simulink model "EcoSIM3_P2_C2_WIP"  (R2014b)
settings: Solver=ode1  SolverMode=SingleTasking  StartTime=0.0  StopTime=4  FixedStep=0.01  RelTol=1e-3
PostLoadFcn:
  | %, if any(exist('dsrtsu_mdlpostloadfcn', 'file') == [2, 3, 6]), try dsrtsu_mdlpostloadfcn('Execute', bdroot); catch fprintf('Error in PostLoadFcn (dsrtsu_mdlpostloadfcn) for model "%s":\n %s\n', bdroot, lasterr); end, end,
InitFcn:
  | tic
  | %Startup_EcoSIM
undefined symbols (not defined in the file or in its folder): canChannel, Controls, DriveCycles, Driver, EM_EFF_MAP, EM_PwrLoss_MAP, EngPwr, EngSpd, EngTrq, Glbl, Overwritten_Mode, Plants, Power, sigbuilder_block, Torque, Trialmap, Veh_Dynamics
libraries: simulink x135, canmsglib x113, fl_lib x104, canlib x89, nesl_utility x56, sdl_lib x29, dspsigops x6, dspswit3 x5, dspstat3 x2, commnoisgen2 x1, dspfdesign x1
(part 15 of 21)

== system EcoSIM3_P2_C2_WIP/Supervisory Controller/Supervisory_IO/VNT Vector/CAN Rx/GCM ==
  Bus Creator7 : BusCreator  Inputs=3
  CAN Receive9 : canlib/CAN Receive  BlockHandle=18097.0002  DeviceMenu=Vector Virtual 1 (Channel 1)  Device=Vector Virtual 1 (Channel 1)  ObjConstructor=canChannel('Vector', 'Virtual 1', 1)  EnableStandardIDsFilter=off  StandardIDs=52  EnableExtendedIDsFilter=off  ExtendedIDs=0  SampleTime=0.01  MsgsPerTimestep=1  StdIDsCombo=Allow only  ExtIDsCombo=Block all  InternalFilterUpdateStatus=on
  CAN Unpack9 : canmsglib/CAN Unpack  CANdbFile=C:\Box Sync\EcoCAR 3\SMS\EcoSIM3_P2_C2\MIL\Final_DBC\EcoCAR3_Controls_Development.dbc  MsgList=GCM_Transmit_MSG052  MsgName=GCM_Transmit_MSG052  MsgIDType=Standard (11-bit identifier)  MsgIdentifier=52  MsgLength=2  SignalInfo=GCM_Heartbeat$2$5$2$2$1$0$1$0$0$31$#GCM_Reported_Gear$13$3$2$1$1$0$1$3$-1$6$#Shift_Complete$1$1$2$2$1$0$1$0$0$1$#charge_mode_request$7$1$2$2$1$0$1$0$0$1$#  NSignals=4  IDPort=off  TimestampPort=off  ErrorPort=off  RemotePort=off  LengthPort=off  StatusPort=off  StartBits=str2num('[int32(2);int32(13);int32(1);int32(7)]')  SignalSizes=str2num('[int32(5);int32(3);int32(1);int32(1)]')  ByteOrders=str2num('[int32(2);int32(2);int32(2);int32(2)]')  DataTypes=str2num('[int32(2);int32(1);int32(2);int32(2)]')  MultiplexTypes=str2num('[int32(1);int32(1);int32(1);int32(1)]')  MultiplexValues=str2num('[double(0);double(0);double(0);double(0)]')  Factors=str2num('[double(1);double(1);double(1);double(1)]')  Offsets=str2num('[double(0);double(3);double(0);double(0)]')  Minimums=str2num('[double(0);double(-1);double(0);double(0)]')  Maximums=str2num('[double(31);double(6);double(1);double(1)]')
      settings: DataFormat=CANdb specified signals
  Terminator10 : Terminator
  FromGCM : Outport
  wires:
  CAN Receive9/2 -> CAN Unpack9/1
  CAN Receive9/1 -> Terminator10/1
  CAN Unpack9/4 -> Bus Creator7/3  "charge_mode_request"
  Bus Creator7/1 -> FromGCM/1  "GCM_CAN_Out"
  CAN Unpack9/3 -> Bus Creator7/2  "Shift_Complete"
  CAN Unpack9/2 -> Bus Creator7/1  "GCM_Reported_Gear"

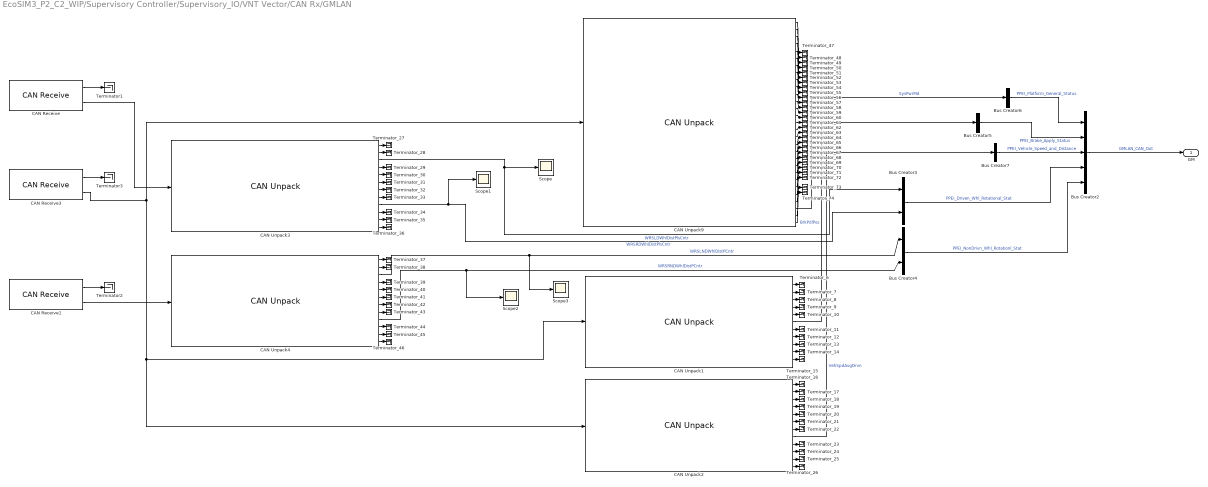
== system EcoSIM3_P2_C2_WIP/Supervisory Controller/Supervisory_IO/VNT Vector/CAN Rx/GMLAN ==
  Bus Creator2 : BusCreator  Inputs=5
  Bus Creator3 : BusCreator  Inputs=2
  Bus Creator4 : BusCreator  Inputs=2
  Bus Creator5 : BusCreator  Inputs=1
  Bus Creator6 : BusCreator  Inputs=1
  Bus Creator7 : BusCreator  Inputs=1
  CAN Receive : canlib/CAN Receive  BlockHandle=18114.0005  DeviceMenu=Kvaser Virtual 1 (Channel 1)  Device=Vector Virtual 1 (Channel 1)  ObjConstructor=canChannel('Vector', 'Virtual 1', 1)  EnableStandardIDsFilter=off  StandardIDs=193  EnableExtendedIDsFilter=off  ExtendedIDs=0  SampleTime=0.01  MsgsPerTimestep=all  StdIDsCombo=Allow only  ExtIDsCombo=Allow all  InternalFilterUpdateStatus=on
  CAN Receive1 : canlib/CAN Receive  BlockHandle=18115.0001  DeviceMenu=Kvaser Virtual 1 (Channel 1)  Device=Vector Virtual 1 (Channel 1)  ObjConstructor=canChannel('Vector', 'Virtual 1', 1)  EnableStandardIDsFilter=off  StandardIDs=197  EnableExtendedIDsFilter=off  ExtendedIDs=0  SampleTime=0.01  MsgsPerTimestep=all  StdIDsCombo=Allow only  ExtIDsCombo=Allow all  InternalFilterUpdateStatus=on
  CAN Receive3 : canlib/CAN Receive  BlockHandle=18116.0001  DeviceMenu=Kvaser Virtual 1 (Channel 1)  Device=Vector Virtual 1 (Channel 1)  ObjConstructor=canChannel('Vector', 'Virtual 1', 1)  EnableStandardIDsFilter=off  StandardIDs=[193 197 241 497 1001]  EnableExtendedIDsFilter=off  ExtendedIDs=0  SampleTime=0.01  MsgsPerTimestep=1  StdIDsCombo=Allow only  ExtIDsCombo=Block all  InternalFilterUpdateStatus=on
  CAN Unpack1 : canmsglib/CAN Unpack  CANdbFile=C:\Users\EcoCAR_HIL\Documents\Khanna\EcoSIM3_P1_0_PHEV_TCU\Final_DBC\GlobalAHS_anon GM CONFIDENTIAL.dbc  MsgList=PPEI_Brake_Apply_Status  MsgName=PPEI_Brake_Apply_Status  MsgIDType=Standard (11-bit identifier)  MsgIdentifier=241  MsgLength=6  SignalInfo=BrkAppSnsrHmPosLrnd$30$1$2$2$1$0$1$0$0$1$#BrkPdlChkData$40$17$2$2$1$0$1$0$0$131071$#BrkPdlInTrvPrt$2$2$2$2$1$0$1$0$0$3$#BrkPdlModTrvl$6$1$2$2$1$0$1$0$0$1$#BrkPdlModTrvlV$7$1$2$2$1$0$1$0$0$1$#BrkPdlPos$8$8$2$2$1$0$3.921570e-01$0$0$1.000000e+02$#BrkPdlPosGrad$16$8$2$1$1$0$40$0$-5120$5080$#BrkPedPosAlvRolngCnt$4$2$2$2$1$0$1$0$0$3$#BrkPedTrvlAchvd$1$1$2$2$1$0$1$0$0$1$#BrkPedTrvlAchvdV$0$1$2$2$1$0$1$0$0$1$#NotEventStat$28$2$2$2$1$0$1$0$0$3$#  NSignals=11  IDPort=off  TimestampPort=off  ErrorPort=off  RemotePort=off  LengthPort=off  StatusPort=off  StartBits=str2num('[int32(30);int32(40);int32(2);int32(6);int32(7);int32(8);int32(16);int32(4);int32(1);int32(0);int32(28)]')  SignalSizes=str2num('[int32(1);int32(17);int32(2);int32(1);int32(1);int32(8);int32(8);int32(2);int32(1);int32(1);int32(2)]')  ByteOrders=str2num('[int32(2);int32(2);int32(2);int32(2);int32(2);int32(2);int32(2);int32(2);int32(2);int32(2);int32(2)]')  DataTypes=str2num('[int32(2);int32(2);int32(2);int32(2);int32(2);int32(2);int32(1);int32(2);int32(2);int32(2);int32(2)]')  MultiplexTypes=str2num('[int32(1);int32(1);int32(1);int32(1);int32(1);int32(1);int32(1);int32(1);int32(1);int32(1);int32(1)]')  MultiplexValues=str2num('[double(0);double(0);double(0);double(0);double(0);double(0);double(0);double(0);double(0);double(0);double(0)]')  Factors=str2num('[double(1);double(1);double(1);double(1);double(1);double(3.921570e-01);double(40);double(1);double(1);double(1);double(1)]')  Offsets=str2num('[double(0);double(0);double(0);double(0);double(0);double(0);double(0);double(0);double(0);double(0);double(0)]')  Minimums=str2num('[double(0);double(0);double(0);double(0);double(0);double(0);double(-5120);double(0);double(0);double(0);double(0)]')  Maximums=str2num('[double(1);double(131071);double(3);double(1);double(1);double(1.000000e+02);double(5080);double(3);double(1);double(1);double(3)]')
      settings: DataFormat=CANdb specified signals
  CAN Unpack2 : canmsglib/CAN Unpack  CANdbFile=C:\Users\EcoCAR_HIL\Documents\Khanna\EcoSIM3_P1_0_PHEV_TCU\Final_DBC\GlobalAHS_anon GM CONFIDENTIAL.dbc  MsgList=PPEI_Vehicle_Speed_and_Distance  MsgName=PPEI_Vehicle_Speed_and_Distance  MsgIDType=Standard (11-bit identifier)  MsgIdentifier=1001  MsgLength=8  SignalInfo=DistRollCntAvgDrvn$24$13$2$2$1$0$1.250000e-01$0$0$1.023875e+03$#DistRollCntAvgDrvnSrc$55$1$2$2$1$0$1$0$0$1$#DistRollCntAvgDrvnV$22$1$2$2$1$0$1$0$0$1$#DstRolCntAvNDrRstOc$53$1$2$2$1$0$1$0$0$1$#DstRolCntAvgDrnRstOc$21$1$2$2$1$0$1$0$0$1$#DstRolCntAvgNonDrvn$56$13$2$2$1$0$1.250000e-01$0$0$1.023875e+03$#DstRolCntAvgNonDrvnV$54$1$2$2$1$0$1$0$0$1$#VehSpdAvgDrvn$8$15$2$2$1$0$1.562500e-02$0$0$5.119844e+02$#VehSpdAvgDrvnSrc$23$1$2$2$1$0$1$0$0$1$#VehSpdAvgDrvnV$7$1$2$2$1$0$1$0$0$1$#VehSpdAvgNDrvn$40$15$2$2$1$0$1.562500e-02$0$0$5.119844e+02$#VehSpdAvgNDrvnV$39$1$2$2$1$0$1$0$0$1$#  NSignals=12  IDPort=off  TimestampPort=off  ErrorPort=off  RemotePort=off  LengthPort=off  StatusPort=off  StartBits=str2num('[int32(24);int32(55);int32(22);int32(53);int32(21);int32(56);int32(54);int32(8);int32(23);int32(7);int32(40);int32(39)]')  SignalSizes=str2num('[int32(13);int32(1);int32(1);int32(1);int32(1);int32(13);int32(1);int32(15);int32(1);int32(1);int32(15);int32(1)]')  ByteOrders=str2num('[int32(2);int32(2);int32(2);int32(2);int32(2);int32(2);int32(2);int32(2);int32(2);int32(2);int32(2);int32(2)]')  DataTypes=str2num('[int32(2);int32(2);int32(2);int32(2);int32(2);int32(2);int32(2);int32(2);int32(2);int32(2);int32(2);int32(2)]')  MultiplexTypes=str2num('[int32(1);int32(1);int32(1);int32(1);int32(1);int32(1);int32(1);int32(1);int32(1);int32(1);int32(1);int32(1)]')  MultiplexValues=str2num('[double(0);double(0);double(0);double(0);double(0);double(0);double(0);double(0);double(0);double(0);double(0);double(0)]')  Factors=str2num('[double(1.250000e-01);double(1);double(1);double(1);double(1);double(1.250000e-01);double(1);double(1.562500e-02);double(1);double(1);double(1.562500e-02);double(1)]')  Offsets=str2num('[double(0);double(0);double(0);double(0);double(0);double(0);double(0);double(0);double(0);double(0);double(0);double(0)]')  Minimums=str2num('[double(0);double(0);double(0);double(0);double(0);double(0);double(0);double(0);double(0);double(0);double(0);double(0)]')  Maximums=str2num('[double(1.023875e+03);double(1);double(1);double(1);double(1);double(1.023875e+03);double(1);double(5.119844e+02);double(1);double(1);double(5.119844e+02);double(1)]')
      settings: DataFormat=CANdb specified signals
  CAN Unpack3 : canmsglib/CAN Unpack  CANdbFile=C:\Users\EcoCAR_HIL\Documents\Khanna\EcoSIM3_P1_0_PHEV_TCU\Final_DBC\GlobalAHS_anon GM CONFIDENTIAL.dbc  MsgList=PPEI_Driven_Whl_Rotational_Stat  MsgName=PPEI_Driven_Whl_Rotational_Stat  MsgIDType=Standard (11-bit identifier)  MsgIdentifier=193  MsgLength=8  SignalInfo=WRSLDSeqNum$4$2$2$2$1$0$1$0$0$3$#WRSLDWhlDisTpRC$6$2$2$2$1$0$1$0$0$3$#WRSLDWhlDistPlsCntr$8$10$2$2$1$0$1$0$0$1023$#WRSLDWhlDistTmstm$24$16$2$2$1$0$1$0$0$65535$#WRSLDWhlDistVal$2$1$2$2$1$0$1$0$0$1$#WRSLDWhlRotStatRst$3$1$2$2$1$0$1$0$0$1$#WRSRDSeqNum$36$2$2$2$1$0$1$0$0$3$#WRSRDWhlDisTpRC$38$2$2$2$1$0$1$0$0$3$#WRSRDWhlDistPlsCntr$40$10$2$2$1$0$1$0$0$1023$#WRSRDWhlDistTmstm$56$16$2$2$1$0$1$0$0$65535$#WRSRDWhlDistVal$34$1$2$2$1$0$1$0$0$1$#WRSRDWhlRotStatRst$35$1$2$2$1$0$1$0$0$1$#  NSignals=12  IDPort=off  TimestampPort=off  ErrorPort=off  RemotePort=off  LengthPort=off  StatusPort=off  StartBits=str2num('[int32(4);int32(6);int32(8);int32(24);int32(2);int32(3);int32(36);int32(38);int32(40);int32(56);int32(34);int32(35)]')  SignalSizes=str2num('[int32(2);int32(2);int32(10);int32(16);int32(1);int32(1);int32(2);int32(2);int32(10);int32(16);int32(1);int32(1)]')  ByteOrders=str2num('[int32(2);int32(2);int32(2);int32(2);int32(2);int32(2);int32(2);int32(2);int32(2);int32(2);int32(2);int32(2)]')  DataTypes=str2num('[int32(2);int32(2);int32(2);int32(2);int32(2);int32(2);int32(2);int32(2);int32(2);int32(2);int32(2);int32(2)]')  MultiplexTypes=str2num('[int32(1);int32(1);int32(1);int32(1);int32(1);int32(1);int32(1);int32(1);int32(1);int32(1);int32(1);int32(1)]')  MultiplexValues=str2num('[double(0);double(0);double(0);double(0);double(0);double(0);double(0);double(0);double(0);double(0);double(0);double(0)]')  Factors=str2num('[double(1);double(1);double(1);double(1);double(1);double(1);double(1);double(1);double(1);double(1);double(1);double(1)]')  Offsets=str2num('[double(0);double(0);double(0);double(0);double(0);double(0);double(0);double(0);double(0);double(0);double(0);double(0)]')  Minimums=str2num('[double(0);double(0);double(0);double(0);double(0);double(0);double(0);double(0);double(0);double(0);double(0);double(0)]')  Maximums=str2num('[double(3);double(3);double(1023);double(65535);double(1);double(1);double(3);double(3);double(1023);double(65535);double(1);double(1)]')
      settings: DataFormat=CANdb specified signals
  CAN Unpack4 : canmsglib/CAN Unpack  CANdbFile=C:\Users\EcoCAR_HIL\Documents\Khanna\EcoSIM3_P1_0_PHEV_TCU\Final_DBC\GlobalAHS_anon GM CONFIDENTIAL.dbc  MsgList=PPEI_NonDrivn_Whl_Rotationl_Stat  MsgName=PPEI_NonDrivn_Whl_Rotationl_Stat  MsgIDType=Standard (11-bit identifier)  MsgIdentifier=197  MsgLength=8  SignalInfo=WRSLNDSeqNum$4$2$2$2$1$0$1$0$0$3$#WRSLNDWhlDisTpRC$6$2$2$2$1$0$1$0$0$3$#WRSLNDWhlDistPCntr$8$10$2$2$1$0$1$0$0$1023$#WRSLNDWhlDistTstm$24$16$2$2$1$0$1$0$0$65535$#WRSLNDWhlDistVal$2$1$2$2$1$0$1$0$0$1$#WRSLNDWhlRotStRst$3$1$2$2$1$0$1$0$0$1$#WRSRNDSeqNum$36$2$2$2$1$0$1$0$0$3$#WRSRNDWhlDisTpRC$38$2$2$2$1$0$1$0$0$3$#WRSRNDWhlDistPCntr$40$10$2$2$1$0$1$0$0$1023$#WRSRNDWhlDistTstm$56$16$2$2$1$0$1$0$0$65535$#WRSRNDWhlDistVal$34$1$2$2$1$0$1$0$0$1$#WRSRNDWhlRotStRst$35$1$2$2$1$0$1$0$0$1$#  NSignals=12  IDPort=off  TimestampPort=off  ErrorPort=off  RemotePort=off  LengthPort=off  StatusPort=off  StartBits=str2num('[int32(4);int32(6);int32(8);int32(24);int32(2);int32(3);int32(36);int32(38);int32(40);int32(56);int32(34);int32(35)]')  SignalSizes=str2num('[int32(2);int32(2);int32(10);int32(16);int32(1);int32(1);int32(2);int32(2);int32(10);int32(16);int32(1);int32(1)]')  ByteOrders=str2num('[int32(2);int32(2);int32(2);int32(2);int32(2);int32(2);int32(2);int32(2);int32(2);int32(2);int32(2);int32(2)]')  DataTypes=str2num('[int32(2);int32(2);int32(2);int32(2);int32(2);int32(2);int32(2);int32(2);int32(2);int32(2);int32(2);int32(2)]')  MultiplexTypes=str2num('[int32(1);int32(1);int32(1);int32(1);int32(1);int32(1);int32(1);int32(1);int32(1);int32(1);int32(1);int32(1)]')  MultiplexValues=str2num('[double(0);double(0);double(0);double(0);double(0);double(0);double(0);double(0);double(0);double(0);double(0);double(0)]')  Factors=str2num('[double(1);double(1);double(1);double(1);double(1);double(1);double(1);double(1);double(1);double(1);double(1);double(1)]')  Offsets=str2num('[double(0);double(0);double(0);double(0);double(0);double(0);double(0);double(0);double(0);double(0);double(0);double(0)]')  Minimums=str2num('[double(0);double(0);double(0);double(0);double(0);double(0);double(0);double(0);double(0);double(0);double(0);double(0)]')  Maximums=str2num('[double(3);double(3);double(1023);double(65535);double(1);double(1);double(3);double(3);double(1023);double(65535);double(1);double(1)]')
      settings: DataFormat=CANdb specified signals
  CAN Unpack9 : canmsglib/CAN Unpack  CANdbFile=C:\Users\EcoCAR_HIL\Documents\Khanna\EcoSIM3_P1_0_PHEV_TCU\Final_DBC\GlobalAHS_anon GM CONFIDENTIAL.dbc  MsgList=PPEI_Platform_General_Status  MsgName=PPEI_Platform_General_Status  MsgIDType=Standard (11-bit identifier)  MsgIdentifier=497  MsgLength=8  SignalInfo=ACCmpsrFldOn$63$1$2$2$1$0$1$0$0$1$#ACCompModReq$11$2$2$2$1$0$1$0$0$3$#ACCompNormLd$48$8$2$2$1$0$1.000000e-01$0$0$2.550000e+01$#ACCompNormLdV$10$1$2$2$1$0$1$0$0$1$#ACCompSysVDA$9$1$2$2$1$0$1$0$0$1$#ACCompSysVDM$60$1$2$2$1$0$1$0$0$1$#AirbgVDA$57$1$2$2$1$0$1$0$0$1$#BkupPwrModeMstrVDA$7$1$2$2$1$0$1$0$0$1$#BkupPwrModeMstrVDM$61$1$2$2$1$0$1$0$0$1$#DispMeasSys$59$1$2$2$1$0$1$0$0$1$#ElvtdIdlCstStReq$32$2$2$2$1$0$1$0$0$3$#EngOilLfRstRq$37$1$2$2$1$0$1$0$0$1$#FuelFltLfRstRqd$56$1$2$2$1$0$1$0$0$1$#ImmblzrPreRelPswdStat$8$1$2$2$1$0$1$0$0$1$#ImmblzrPreRelPswrd$24$16$2$2$1$0$1$0$0$65535$#PMMAccTrmSt$2$1$2$2$1$0$1$0$0$1$#PMMRunCrkTrmSt$3$1$2$2$1$0$1$0$0$1$#PTORSMstrEngShtReq$13$1$2$2$1$0$1$0$0$1$#PTORmStMsEngStRq$14$1$2$2$1$0$1$0$0$1$#PrkBrkSwAtv$36$1$2$2$1$0$1$0$0$1$#PrkBrkVDA$35$1$2$2$1$0$1$0$0$1$#PrkBrkVDM$62$1$2$2$1$0$1$0$0$1$#RmVehStrRq$15$1$2$2$1$0$1$0$0$1$#SIRDpl$58$1$2$2$1$0$1$0$0$1$#SysBkUpPwrMd$4$2$2$2$1$0$1$0$0$3$#SysBkupPwrMdEn$6$1$2$2$1$0$1$0$0$1$#SysPwrMd$0$2$2$2$1$0$1$0$0$3$#ThrtlPrgrsnReq$38$2$2$2$1$0$1$0$0$3$#TrStLgMdAtv$34$1$2$2$1$0$1$0$0$1$#  NSignals=29  IDPort=off  TimestampPort=off  ErrorPort=off  RemotePort=off  LengthPort=off  StatusPort=off  StartBits=str2num('[int32(63);int32(11);int32(48);int32(10);int32(9);int32(60);int32(57);int32(7);int32(61);int32(59);int32(32);int32(37);int32(56);int32(8);int32(24);int32(2);int32(3);int32(13);int32(14);int32(36);int32(35);int32(62);int32(15);int32(58);int32(4);int32(6);int32(0);int32(38);int32(34)]')  SignalSizes=str2num('[int32(1);int32(2);int32(8);int32(1);int32(1);int32(1);int32(1);int32(1);int32(1);int32(1);int32(2);int32(1);int32(1);int32(1);int32(16);int32(1);int32(1);int32(1);int32(1);int32(1);int32(1);int32(1);int32(1);int32(1);int32(2);int32(1);int32(2);int32(2);int32(1)]')  ByteOrders=str2num('[int32(2);int32(2);int32(2);int32(2);int32(2);int32(2);int32(2);int32(2);int32(2);int32(2);int32(2);int32(2);int32(2);int32(2);int32(2);int32(2);int32(2);int32(2);int32(2);int32(2);int32(2);int32(2);int32(2);int32(2);int32(2);int32(2);int32(2);int32(2);int32(2)]')  DataTypes=str2num('[int32(2);int32(2);int32(2);int32(2);int32(2);int32(2);int32(2);int32(2);int32(2);int32(2);int32(2);int32(2);int32(2);int32(2);int32(2);int32(2);int32(2);int32(2);int32(2);int32(2);int32(2);int32(2);int32(2);int32(2);int32(2);int32(2);int32(2);int32(2);int32(2)]')  MultiplexTypes=str2num('[int32(1);int32(1);int32(1);int32(1);int32(1);int32(1);int32(1);int32(1);int32(1);int32(1);int32(1);int32(1);int32(1);int32(1);int32(1);int32(1);int32(1);int32(1);int32(1);int32(1);int32(1);int32(1);int32(1);int32(1);int32(1);int32(1);int32(1);int32(1);int32(1)]')  MultiplexValues=str2num('[double(0);double(0);double(0);double(0);double(0);double(0);double(0);double(0);double(0);double(0);double(0);double(0);double(0);double(0);double(0);double(0);double(0);double(0);double(0);double(0);double(0);double(0);double(0);double(0);double(0);double(0);double(0);double(0);double(0)]')  Factors=str2num('[double(1);double(1);double(1.000000e-01);double(1);double(1);double(1);double(1);double(1);double(1);double(1);double(1);double(1);double(1);double(1);double(1);double(1);double(1);double(1);double(1);double(1);double(1);double(1);double(1);double(1);double(1);double(1);double(1);double(1);double(1)]')  Offsets=str2num('[double(0);double(0);double(0);double(0);double(0);double(0);double(0);double(0);double(0);double(0);double(0);double(0);double(0);double(0);double(0);double(0);double(0);double(0);double(0);double(0);double(0);double(0);double(0);double(0);double(0);double(0);double(0);double(0);double(0)]')  Minimums=str2num('[double(0);double(0);double(0);double(0);double(0);double(0);double(0);double(0);double(0);double(0);double(0);double(0);double(0);double(0);double(0);double(0);double(0);double(0);double(0);double(0);double(0);double(0);double(0);double(0);double(0);double(0);double(0);double(0);double(0)]')  Maximums=str2num('[double(1);double(3);double(2.550000e+01);double(1);double(1);double(1);double(1);double(1);double(1);double(1);double(3);double(1);double(1);double(1);double(65535);double(1);double(1);double(1);double(1);double(1);double(1);double(1);double(1);double(1);double(3);double(1);double(3);double(3);double(1)]')
      settings: DataFormat=CANdb specified signals
  Scope{,1..3} (4 alike) : Scope
      Scope settings: TimeRange=20  YMin=0  YMax=3  SaveName=ScopeData19
      Scope1 settings: TimeRange=20  YMin=0  YMax=3  SaveName=ScopeData5
      Scope2 settings: TimeRange=20  YMin=0  YMax=3  SaveName=ScopeData15
      Scope3 settings: TimeRange=20  YMin=0  YMax=3  SaveName=ScopeData24
  Terminator1 : Terminator
  Terminator2 : Terminator
  Terminator3 : Terminator
  Terminator_{6..74} (69 alike) : Terminator
  GM : Outport
  wires:
  CAN Unpack4/3 -> Scope3/1, Bus Creator4/1  "WRSLNDWhlDistPCntr"
  CAN Unpack3/3 -> Bus Creator3/1, Scope/1  "WRSLDWhlDistPlsCntr"
  Bus Creator4/1 -> Bus Creator2/5  "PPEI_NonDrivn_Whl_Rotationl_Stat"
  Bus Creator3/1 -> Bus Creator2/4  "PPEI_Driven_Whl_Rotational_Stat"
  CAN Unpack4/9 -> Scope2/1, Bus Creator4/2  "WRSRNDWhlDistPCntr"
  CAN Unpack3/9 -> Scope1/1, Bus Creator3/2  "WRSRDWhlDistPlsCntr"
  Bus Creator2/1 -> GM/1  "GMLAN_CAN_Out"
  Bus Creator5/1 -> Bus Creator2/2  "PPEI_Brake_Apply_Status"
  Bus Creator6/1 -> Bus Creator2/1  "PPEI_Platform_General_Status"
  CAN Unpack2/8 -> Bus Creator7/1  "VehSpdAvgDrvn"
  Bus Creator7/1 -> Bus Creator2/3  "PPEI_Vehicle_Speed_and_Distance"
  CAN Unpack1/6 -> Bus Creator5/1  "BrkPdlPos"
  CAN Unpack9/27 -> Bus Creator6/1  "SysPwrMd"
  CAN Receive3/2 -> CAN Unpack9/1, CAN Unpack2/1, CAN Unpack1/1
  CAN Receive3/1 -> Terminator3/1
  CAN Unpack1/1 -> Terminator_6/1
  CAN Unpack1/2 -> Terminator_7/1
  CAN Unpack1/3 -> Terminator_8/1
  CAN Unpack1/4 -> Terminator_9/1
  CAN Unpack1/5 -> Terminator_10/1
  CAN Unpack1/7 -> Terminator_11/1
  CAN Unpack1/8 -> Terminator_12/1
  CAN Unpack1/9 -> Terminator_13/1
  CAN Unpack1/10 -> Terminator_14/1
  CAN Unpack1/11 -> Terminator_15/1
  CAN Unpack2/1 -> Terminator_16/1
  CAN Unpack2/2 -> Terminator_17/1
  CAN Unpack2/3 -> Terminator_18/1
  CAN Unpack2/4 -> Terminator_19/1
  CAN Unpack2/5 -> Terminator_20/1
  CAN Unpack2/6 -> Terminator_21/1
  CAN Unpack2/7 -> Terminator_22/1
  CAN Unpack2/9 -> Terminator_23/1
  CAN Unpack2/10 -> Terminator_24/1
  CAN Unpack2/11 -> Terminator_25/1
  CAN Unpack2/12 -> Terminator_26/1
  CAN Unpack3/1 -> Terminator_27/1
  CAN Unpack3/2 -> Terminator_28/1
  CAN Unpack3/4 -> Terminator_29/1
  CAN Unpack3/5 -> Terminator_30/1
  CAN Unpack3/6 -> Terminator_31/1
  CAN Unpack3/7 -> Terminator_32/1
  CAN Unpack3/8 -> Terminator_33/1
  CAN Unpack3/10 -> Terminator_34/1
  CAN Unpack3/11 -> Terminator_35/1
  CAN Unpack3/12 -> Terminator_36/1
  CAN Unpack4/1 -> Terminator_37/1
  CAN Unpack4/2 -> Terminator_38/1
  CAN Unpack4/4 -> Terminator_39/1
  CAN Unpack4/5 -> Terminator_40/1
  CAN Unpack4/6 -> Terminator_41/1
  CAN Unpack4/7 -> Terminator_42/1
  CAN Unpack4/8 -> Terminator_43/1
  CAN Unpack4/10 -> Terminator_44/1
  CAN Unpack4/11 -> Terminator_45/1
  CAN Unpack4/12 -> Terminator_46/1
  CAN Unpack9/1 -> Terminator_47/1
  CAN Unpack9/2 -> Terminator_48/1
  CAN Unpack9/3 -> Terminator_49/1
  CAN Unpack9/4 -> Terminator_50/1
  CAN Unpack9/5 -> Terminator_51/1
  CAN Unpack9/6 -> Terminator_52/1
  CAN Unpack9/7 -> Terminator_53/1
  CAN Unpack9/8 -> Terminator_54/1
  CAN Unpack9/9 -> Terminator_55/1
  CAN Unpack9/10 -> Terminator_56/1
  CAN Unpack9/11 -> Terminator_57/1
  CAN Unpack9/12 -> Terminator_58/1
  CAN Unpack9/13 -> Terminator_59/1
  CAN Unpack9/14 -> Terminator_60/1
  CAN Unpack9/15 -> Terminator_61/1
  CAN Unpack9/16 -> Terminator_62/1
  CAN Unpack9/17 -> Terminator_63/1
  CAN Unpack9/18 -> Terminator_64/1
  CAN Unpack9/19 -> Terminator_65/1
  CAN Unpack9/20 -> Terminator_66/1
  CAN Unpack9/21 -> Terminator_67/1
  CAN Unpack9/22 -> Terminator_68/1
  CAN Unpack9/23 -> Terminator_69/1
  CAN Unpack9/24 -> Terminator_70/1
  CAN Unpack9/25 -> Terminator_71/1
  CAN Unpack9/26 -> Terminator_72/1
  CAN Unpack9/28 -> Terminator_73/1
  CAN Unpack9/29 -> Terminator_74/1
  CAN Receive/1 -> Terminator1/1
  CAN Receive/2 -> CAN Unpack3/1
  CAN Receive1/2 -> CAN Unpack4/1
  CAN Receive1/1 -> Terminator2/1

== system EcoSIM3_P2_C2_WIP/Supervisory Controller/Supervisory_IO/VNT Vector/CAN Tx/BAS ==
  BAS : Inport
  CAN Transmit1 : canlib/CAN Transmit  BlockHandle=18313.0001  DeviceMenu=(none)  Device=Vector Virtual 1 (Channel 1)  ObjConstructor=canChannel('Vector', 'Virtual 1', 1)  EnablePeriodicTransmit=off  MessagePeriod=1.000
  Mux : Mux  Inputs=2
  SetLimits : Subsystem
  SetValues : Subsystem
  wires:
  BAS/1 -> SetValues/1(In1), SetLimits/1(In1)
  SetValues/1(Out1) -> CAN Transmit1/1
  SetLimits/1(Out1) -> Mux/1

== system EcoSIM3_P2_C2_WIP/Supervisory Controller/Supervisory_IO/VNT Vector/CAN Tx/ESS ==
  ESS : Inport
  Bus Selector2 : BusSelector  OutputSignals=ESS_Signals_A123.hsc_bcm_enable,ESS_Signals_A123.hsc_bcm_epo,ESS_Signals_A123.hsc_bcm_leakage_ena,ESS_Signals_A123.hsc_bcm_mainc_close
  CAN Pack4 : canmsglib/CAN Pack  CANdbFile=C:\Users\EcoCAR_HIL\Documents\Khanna\EcoSIM3_P1_0_PHEV_TCU\Final_DBC\BCM_VehBus_Std.dbc  MsgList=BCM_Request  MsgName=BCM_Request  MsgIDType=Standard (11-bit identifier)  MsgIdentifier=1024  MsgLength=4  SignalInfo=hsc_bcm_enable$0$1$2$2$1$0$1$0$0$1$#hsc_bcm_epo$1$1$2$2$1$0$1$0$0$1$#hsc_bcm_leakage_ena$3$1$2$2$1$0$1$0$0$1$#hsc_bcm_mainc_close$2$1$2$2$1$0$1$0$0$1$#  NSignals=4  StartBits=str2num('[int32(0);int32(1);int32(3);int32(2)]')  SignalSizes=str2num('[int32(1);int32(1);int32(1);int32(1)]')  ByteOrders=str2num('[int32(2);int32(2);int32(2);int32(2)]')  DataTypes=str2num('[int32(2);int32(2);int32(2);int32(2)]')  MultiplexTypes=str2num('[int32(1);int32(1);int32(1);int32(1)]')  MultiplexValues=str2num('[double(0);double(0);double(0);double(0)]')  Factors=str2num('[double(1);double(1);double(1);double(1)]')  Offsets=str2num('[double(0);double(0);double(0);double(0)]')  Minimums=str2num('[double(0);double(0);double(0);double(0)]')  Maximums=str2num('[double(1);double(1);double(1);double(1)]')  Remote=off
      settings: DataFormat=CANdb specified signals
  CAN Transmit4 : canlib/CAN Transmit  BlockHandle=18375.0001  DeviceMenu=Vector Virtual 1 (Channel 1)  Device=Vector Virtual 1 (Channel 1)  ObjConstructor=canChannel('Vector', 'Virtual 1', 1)  EnablePeriodicTransmit=off  MessagePeriod=1.000
  Rate Transition{,1..3} (4 alike) : RateTransition
  wires:
  ESS/1 -> Bus Selector2/1
  Bus Selector2/2 -> Rate Transition1/1  "<hsc_bcm_epo>"
  Bus Selector2/3 -> Rate Transition2/1  "<hsc_bcm_leakage_ena>"
  CAN Pack4/1 -> CAN Transmit4/1
  Bus Selector2/4 -> Rate Transition3/1  "<hsc_bcm_mainc_close>"
  Bus Selector2/1 -> Rate Transition/1  "<hsc_bcm_enable>"
  Rate Transition/1 -> CAN Pack4/1
  Rate Transition1/1 -> CAN Pack4/2
  Rate Transition2/1 -> CAN Pack4/3
  Rate Transition3/1 -> CAN Pack4/4

== system EcoSIM3_P2_C2_WIP/Supervisory Controller/Supervisory_IO/VNT Vector/CAN Tx/Electric Motor ==
  EMTransmit : Inport
  Bus Selector : BusSelector  OutputSignals=Rotation_Direction,Inverter_Enable,Torque_Command
  Bus Selector1 : BusSelector  OutputSignals=EM_Messages_Rhinehart
  CAN Pack : canmsglib/CAN Pack  CANdbFile=C:\Users\EcoCAR_HIL\Documents\Khanna\EcoSIM3_P1_0_PHEV_TCU\Final_DBC\20160113 RMS PM CAN DB.dbc  MsgList=M192_Command_Message  MsgName=M192_Command_Message  MsgIDType=Standard (11-bit identifier)  MsgIdentifier=192  MsgLength=8  SignalInfo=Direction_Command$32$1$1$2$1$0$1$0$0$1$#Inverter_Discharge$41$1$1$2$1$0$1$0$0$1$#Inverter_Enable$40$1$1$2$1$0$1$0$0$1$#Speed_Command$16$16$1$1$1$0$1$0$-32768$32767$#Speed_Mode_Enable$42$1$1$2$1$0$1$0$0$1$#Torque_Command$0$16$1$1$1$0$1.000000e-01$0$-3.276800e+03$3.276700e+03$#Torque_Limit_Command$48$16$1$1$1$0$1$0$-3.276800e+03$3.276700e+03$#  NSignals=7  StartBits=str2num('[int32(32);int32(41);int32(40);int32(16);int32(42);int32(0);int32(48)]')  SignalSizes=str2num('[int32(1);int32(1);int32(1);int32(16);int32(1);int32(16);int32(16)]')  ByteOrders=str2num('[int32(1);int32(1);int32(1);int32(1);int32(1);int32(1);int32(1)]')  DataTypes=str2num('[int32(2);int32(2);int32(2);int32(1);int32(2);int32(1);int32(1)]')  MultiplexTypes=str2num('[int32(1);int32(1);int32(1);int32(1);int32(1);int32(1);int32(1)]')  MultiplexValues=str2num('[double(0);double(0);double(0);double(0);double(0);double(0);double(0)]')  Factors=str2num('[double(1);double(1);double(1);double(1);double(1);double(1.000000e-01);double(1)]')  Offsets=str2num('[double(0);double(0);double(0);double(0);double(0);double(0);double(0)]')  Minimums=str2num('[double(0);double(0);double(0);double(-32768);double(0);double(-3.276800e+03);double(-3.276800e+03)]')  Maximums=str2num('[double(1);double(1);double(1);double(32767);double(1);double(3.276700e+03);double(3.276700e+03)]')  Remote=off
      settings: DataFormat=CANdb specified signals
  CAN Transmit : canlib/CAN Transmit  BlockHandle=18395.0001  DeviceMenu=Vector Virtual 1 (Channel 1)  Device=Vector Virtual 1 (Channel 2)  ObjConstructor=canChannel('Vector', 'Virtual 1', 2)  EnablePeriodicTransmit=off  MessagePeriod=1.000
  Ground_{1..4} (4 alike) : Ground
  Rate Transition : RateTransition
  Rate Transition1 : RateTransition
  Rate Transition2 : RateTransition
  wires:
  EMTransmit/1 -> Bus Selector1/1
  Bus Selector/2 -> Rate Transition1/1  "<Inverter_Enable>"
  Bus Selector/3 -> Rate Transition2/1  "<Torque_Command>"
  Bus Selector/1 -> Rate Transition/1  "<Rotation_Direction>"
  CAN Pack/1 -> CAN Transmit/1
  Bus Selector1/1 -> Bus Selector/1  "<EM_Messages_Rhinehart>"
  Rate Transition/1 -> CAN Pack/1
  Rate Transition1/1 -> CAN Pack/3
  Rate Transition2/1 -> CAN Pack/6
  Ground_1/1 -> CAN Pack/2
  Ground_2/1 -> CAN Pack/4
  Ground_3/1 -> CAN Pack/5
  Ground_4/1 -> CAN Pack/7

== system EcoSIM3_P2_C2_WIP/Supervisory Controller/Supervisory_IO/VNT Vector/CAN Tx/ICE_BAS_Trans ==
  ICE_BAS_Trans : Inport
  Bus Selector1 : BusSelector  OutputSignals=Engine_Messages.ICE_Torque_Request_Nm,Engine_Messages.Engine_Run,Engine_Messages.Engine_On,Trans_Receive.Shift_Request,Trans_Receive.Gear_Request,GCM_Messages_Transmission.Clutch_Status,GCM_Messages_Transmission.GCM_Gear_Request,CP1_Messages.MSG_HYB_01.MY01_SleepAckn,CP1_Messages.MSG_HYB_15.MY15_CCU_posDes
  CAN Pack1 : canmsglib/CAN Pack  CANdbFile=C:\Users\EcoCAR_HIL\Box Sync\EcoCAR 3\SMS\EcoSIM3_P2_C2\MIL\Final_DBC\Engine_Transmission_BAS.dbc  MsgList=ECO_Engine_MSG101  MsgName=ECO_Engine_MSG101  MsgIDType=Standard (11-bit identifier)  MsgIdentifier=101  MsgLength=3  SignalInfo=ICE_Torque_Request_Nm$9$15$2$2$1$0$1.000000e-02$0$0$3.276700e+02$#ISP_R$8$1$2$2$1$0$1$0$0$1$#PCM_Wake$23$1$2$2$1$0$1$0$0$1$#  NSignals=3  StartBits=str2num('[int32(9);int32(8);int32(23)]')  SignalSizes=str2num('[int32(15);int32(1);int32(1)]')  ByteOrders=str2num('[int32(2);int32(2);int32(2)]')  DataTypes=str2num('[int32(2);int32(2);int32(2)]')  MultiplexTypes=str2num('[int32(1);int32(1);int32(1)]')  MultiplexValues=str2num('[double(0);double(0);double(0)]')  Factors=str2num('[double(1.000000e-02);double(1);double(1)]')  Offsets=str2num('[double(0);double(0);double(0)]')  Minimums=str2num('[double(0);double(0);double(0)]')  Maximums=str2num('[double(3.276700e+02);double(1);double(1)]')  Remote=off
      settings: DataFormat=CANdb specified signals
  CAN Pack2 : canmsglib/CAN Pack  CANdbFile=C:\Box Sync\EcoCAR 3\SMS\EcoSIM3_P2_C2\MIL\Final_DBC\EcoCAR3_Controls_Development.dbc  MsgList=GCM_Receive_MSG095  MsgName=GCM_Receive_MSG095  MsgIDType=Standard (11-bit identifier)  MsgIdentifier=95  MsgLength=2  SignalInfo=BAS_Relay_Close$7$1$2$2$1$0$1$0$0$1$#BCM_Relay_Close$6$1$2$2$1$0$1$0$0$1$#Clutch_Status$14$2$2$2$1$0$1$0$0$3$#ECM_Relay_Close$5$1$2$2$1$0$1$0$0$1$#EM_Relay_Close$4$1$2$2$1$0$1$0$0$1$#GCM_Gear_Request$1$3$2$1$1$0$1$3$-1$6$#  NSignals=6  StartBits=str2num('[int32(7);int32(6);int32(14);int32(5);int32(4);int32(1)]')  SignalSizes=str2num('[int32(1);int32(1);int32(2);int32(1);int32(1);int32(3)]')  ByteOrders=str2num('[int32(2);int32(2);int32(2);int32(2);int32(2);int32(2)]')  DataTypes=str2num('[int32(2);int32(2);int32(2);int32(2);int32(2);int32(1)]')  MultiplexTypes=str2num('[int32(1);int32(1);int32(1);int32(1);int32(1);int32(1)]')  MultiplexValues=str2num('[double(0);double(0);double(0);double(0);double(0);double(0)]')  Factors=str2num('[double(1);double(1);double(1);double(1);double(1);double(1)]')  Offsets=str2num('[double(0);double(0);double(0);double(0);double(0);double(3)]')  Minimums=str2num('[double(0);double(0);double(0);double(0);double(0);double(-1)]')  Maximums=str2num('[double(1);double(1);double(3);double(1);double(1);double(6)]')  Remote=off
      settings: DataFormat=CANdb specified signals
  CAN Pack3 : canmsglib/CAN Pack  CANdbFile=C:\Users\EcoCAR_HIL\Documents\Khanna\EcoSIM3_P1_0_PHEV_TCU\Final_DBC\Engine_Transmission_BAS.dbc  MsgList=ECO_Trans_Receive_MSG105  MsgName=ECO_Trans_Receive_MSG105  MsgIDType=Standard (11-bit identifier)  MsgIdentifier=105  MsgLength=1  SignalInfo=Clutch_Request$4$1$2$2$1$0$1$0$0$1$#Gear_Request$5$3$2$2$1$0$1$0$0$7$#  NSignals=2  StartBits=str2num('[int32(4);int32(5)]')  SignalSizes=str2num('[int32(1);int32(3)]')  ByteOrders=str2num('[int32(2);int32(2)]')  DataTypes=str2num('[int32(2);int32(2)]')  MultiplexTypes=str2num('[int32(1);int32(1)]')  MultiplexValues=str2num('[double(0);double(0)]')  Factors=str2num('[double(1);double(1)]')  Offsets=str2num('[double(0);double(0)]')  Minimums=str2num('[double(0);double(0)]')  Maximums=str2num('[double(1);double(7)]')  Remote=off
      settings: DataFormat=CANdb specified signals
  CAN Pack4 : canmsglib/CAN Pack  CANdbFile=C:\Box Sync\EcoCAR 3\SMS\EcoSIM3_P2_C2\MIL\Final_DBC\FTE_ElecHydAct.dbc  MsgList=MSG_HYB_01  MsgName=MSG_HYB_01  MsgIDType=Standard (11-bit identifier)  MsgIdentifier=934  MsgLength=8  SignalInfo=MY01_Checksum$0$8$1$2$1$0$1$0$-Inf$Inf$#MY01_Counter$8$4$1$2$1$0$1$0$0$15$#MY01_SleepAckn$12$1$1$2$1$0$1$0$-Inf$Inf$#  NSignals=3  StartBits=str2num('[int32(0);int32(8);int32(12)]')  SignalSizes=str2num('[int32(8);int32(4);int32(1)]')  ByteOrders=str2num('[int32(1);int32(1);int32(1)]')  DataTypes=str2num('[int32(2);int32(2);int32(2)]')  MultiplexTypes=str2num('[int32(1);int32(1);int32(1)]')  MultiplexValues=str2num('[double(0);double(0);double(0)]')  Factors=str2num('[double(1);double(1);double(1)]')  Offsets=str2num('[double(0);double(0);double(0)]')  Minimums=str2num('[double(-Inf);double(0);double(-Inf)]')  Maximums=str2num('[double(Inf);double(15);double(Inf)]')  Remote=off
      settings: DataFormat=CANdb specified signals
  CAN Pack5 : canmsglib/CAN Pack  CANdbFile=C:\Box Sync\EcoCAR 3\SMS\EcoSIM3_P2_C2\MIL\Final_DBC\FTE_ElecHydAct.dbc  MsgList=MSG_HYB_15  MsgName=MSG_HYB_15  MsgIDType=Standard (11-bit identifier)  MsgIdentifier=150  MsgLength=8  SignalInfo=MY15_CCU_pLimReq$15$1$1$2$1$0$1$0$-Inf$Inf$#MY15_CCU_pMax$20$4$1$2$1$0$1$0$-Inf$Inf$#MY15_CCU_pMin$16$4$1$2$1$0$1$0$-Inf$Inf$#MY15_CCU_posDes$24$13$1$2$1$0$1$0$0$6327$#MY15_CCU_stModeReq$12$3$1$2$1$0$1$0$-Inf$Inf$#MY15_Checksum$0$8$1$2$1$0$1$0$-Inf$Inf$#MY15_Counter$8$4$1$2$1$0$1$0$-Inf$Inf$#  NSignals=7  StartBits=str2num('[int32(15);int32(20);int32(16);int32(24);int32(12);int32(0);int32(8)]')  SignalSizes=str2num('[int32(1);int32(4);int32(4);int32(13);int32(3);int32(8);int32(4)]')  ByteOrders=str2num('[int32(1);int32(1);int32(1);int32(1);int32(1);int32(1);int32(1)]')  DataTypes=str2num('[int32(2);int32(2);int32(2);int32(2);int32(2);int32(2);int32(2)]')  MultiplexTypes=str2num('[int32(1);int32(1);int32(1);int32(1);int32(1);int32(1);int32(1)]')  MultiplexValues=str2num('[double(0);double(0);double(0);double(0);double(0);double(0);double(0)]')  Factors=str2num('[double(1);double(1);double(1);double(1);double(1);double(1);double(1)]')  Offsets=str2num('[double(0);double(0);double(0);double(0);double(0);double(0);double(0)]')  Minimums=str2num('[double(-Inf);double(-Inf);double(-Inf);double(0);double(-Inf);double(-Inf);double(-Inf)]')  Maximums=str2num('[double(Inf);double(Inf);double(Inf);double(6327);double(Inf);double(Inf);double(Inf)]')  Remote=off
      settings: DataFormat=CANdb specified signals
  CAN Transmit3 : canlib/CAN Transmit  BlockHandle=18424.0001  DeviceMenu=Vector Virtual 1 (Channel 1)  Device=Vector Virtual 1 (Channel 1)  ObjConstructor=canChannel('Vector', 'Virtual 1', 1)  EnablePeriodicTransmit=off  MessagePeriod=1.000
  Ground_{1..4} (4 alike) : Ground
  Mux : Mux  Inputs=5
  Rate Transition{,1..8} (9 alike) : RateTransition
  Scope : Scope
      settings: SaveName=ScopeData64
  wires:
  ICE_BAS_Trans/1 -> Bus Selector1/1
  Bus Selector1/5 -> Rate Transition3/1  "<Gear_Request>"
  Bus Selector1/1 -> Rate Transition/1  "<ICE_Torque_Request_Nm>"
  Rate Transition/1 -> CAN Pack1/1
  Rate Transition3/1 -> CAN Pack3/2
  Bus Selector1/2 -> Rate Transition4/1  "<Engine_Run>"
  Bus Selector1/3 -> Rate Transition5/1  "<Engine_On>"
  Rate Transition4/1 -> CAN Pack1/2
  Rate Transition5/1 -> CAN Pack1/3
  Bus Selector1/4 -> Rate Transition1/1  "<Shift_Request>"
  Rate Transition1/1 -> CAN Pack3/1
  Bus Selector1/6 -> Rate Transition2/1  "<Clutch_Status>"
  Rate Transition2/1 -> CAN Pack2/3
  Bus Selector1/7 -> Rate Transition6/1  "<GCM_Gear_Request>"
  Rate Transition6/1 -> Scope/1, CAN Pack2/6
  Ground_1/1 -> CAN Pack2/1
  Ground_2/1 -> CAN Pack2/2
  Ground_3/1 -> CAN Pack2/4
  Ground_4/1 -> CAN Pack2/5
  Mux/1 -> CAN Transmit3/1
  Rate Transition7/1 -> CAN Pack4/3
  Bus Selector1/8 -> Rate Transition7/1  "<MY01_SleepAckn>"
  Bus Selector1/9 -> Rate Transition8/1  "<MY15_CCU_posDes>"
  Rate Transition8/1 -> CAN Pack5/4
  CAN Pack5/1 -> Mux/5
  CAN Pack4/1 -> Mux/4
  CAN Pack2/1 -> Mux/3
  CAN Pack3/1 -> Mux/2
  CAN Pack1/1 -> Mux/1

== system EcoSIM3_P2_C2_WIP/Supervisory Controller/Supervisory_IO/VNT Vector/CAN Tx/MABx-DCDC ==
  MABx : Inport
  Bus Selector1 : BusSelector  OutputSignals=DC_DC.LowVoltEnblRq,DC_DC.LwVltStpntCmnd,DC_DC.PrplsnSysAtv
  Bus Selector3 : BusSelector  OutputSignals=Supervisory.Mode,GCM_Messages_Transmission.Shift_In_Progress
  CAN Pack1 : canmsglib/CAN Pack  CANdbFile=C:\Box Sync\EcoCAR 3\SMS\EcoSIM3_P2_C2\MIL\Final_DBC\GlobalA_v4p3_APM_PE_v2.dbc  MsgList=PTEI_Hybrid_General_Status_1  MsgName=PTEI_Hybrid_General_Status_1  MsgIDType=Standard (11-bit identifier)  MsgIdentifier=468  MsgLength=2  SignalInfo=HybContClrLgsDiag$6$1$2$2$1$0$1$0$0$1$#LowVoltEnblRq$7$1$2$2$1$0$1$0$0$1$#LwVltStpntCmnd$8$8$2$2$1$0$7.843140e-02$0$0$2.000001e+01$#PrplsnSysAtv$5$1$2$2$1$0$1$0$0$1$#  NSignals=4  StartBits=str2num('[int32(6);int32(7);int32(8);int32(5)]')  SignalSizes=str2num('[int32(1);int32(1);int32(8);int32(1)]')  ByteOrders=str2num('[int32(2);int32(2);int32(2);int32(2)]')  DataTypes=str2num('[int32(2);int32(2);int32(2);int32(2)]')  MultiplexTypes=str2num('[int32(1);int32(1);int32(1);int32(1)]')  MultiplexValues=str2num('[double(0);double(0);double(0);double(0)]')  Factors=str2num('[double(1);double(1);double(7.843140e-02);double(1)]')  Offsets=str2num('[double(0);double(0);double(0);double(0)]')  Minimums=str2num('[double(0);double(0);double(0);double(0)]')  Maximums=str2num('[double(1);double(1);double(2.000001e+01);double(1)]')  Remote=off
      settings: DataFormat=CANdb specified signals
  CAN Pack5 : canmsglib/CAN Pack  CANdbFile=C:\Box Sync\EcoCAR 3\SMS\EcoSIM3_P2_C2\MIL\Final_DBC\EcoCAR3_Controls_Development.dbc  MsgList=MABx_Transmit_MSG094  MsgName=MABx_Transmit_MSG094  MsgIDType=Standard (11-bit identifier)  MsgIdentifier=94  MsgLength=4  SignalInfo=Charge_Sustain_Switch$23$1$2$2$1$0$1$0$0$1$#Charging_Complete$11$1$2$2$1$0$1$0$0$1$#Charging_Light$10$1$2$2$1$0$1$0$0$1$#EPB_Disengage_Pulse$16$1$2$2$1$0$1$0$0$1$#EPB_Engage_Pulse$17$1$2$2$1$0$1$0$0$1$#Eng_Fuel_Pump$19$1$2$2$1$0$1$0$0$1$#Eng_Fusebox$18$1$2$2$1$0$1$0$0$1$#Engine_On_Switch$22$1$2$2$1$0$1$0$0$1$#GFD_Light$9$1$2$2$1$0$1$0$0$1$#MABx_Heartbeat$2$5$2$2$1$0$1$0$0$31$#Mode$7$1$2$2$1$0$1$0$0$1$#PRNDL$29$3$2$2$1$0$1$0$0$5$#Regen_Disable_Switch$21$1$2$2$1$0$1$0$0$1$#Shift_In_Progress$28$1$2$2$1$0$1$0$0$1$#Shutdown_Complete$20$1$2$2$1$0$1$0$0$1$#Starter_Request$0$1$2$2$1$0$1$0$0$1$#Veh_Relay_Request$1$1$2$2$1$0$1$0$0$1$#Vehicle_Mode$12$4$2$2$1$0$1$0$0$15$#Vehicle_Ready_Light$8$1$2$2$1$0$1$0$0$1$#  NSignals=19  StartBits=str2num('[int32(23);int32(11);int32(10);int32(16);int32(17);int32(19);int32(18);int32(22);int32(9);int32(2);int32(7);int32(29);int32(21);int32(28);int32(20);int32(0);int32(1);int32(12);int32(8)]')  SignalSizes=str2num('[int32(1);int32(1);int32(1);int32(1);int32(1);int32(1);int32(1);int32(1);int32(1);int32(5);int32(1);int32(3);int32(1);int32(1);int32(1);int32(1);int32(1);int32(4);int32(1)]')  ByteOrders=str2num('[int32(2);int32(2);int32(2);int32(2);int32(2);int32(2);int32(2);int32(2);int32(2);int32(2);int32(2);int32(2);int32(2);int32(2);int32(2);int32(2);int32(2);int32(2);int32(2)]')  DataTypes=str2num('[int32(2);int32(2);int32(2);int32(2);int32(2);int32(2);int32(2);int32(2);int32(2);int32(2);int32(2);int32(2);int32(2);int32(2);int32(2);int32(2);int32(2);int32(2);int32(2)]')  MultiplexTypes=str2num('[int32(1);int32(1);int32(1);int32(1);int32(1);int32(1);int32(1);int32(1);int32(1);int32(1);int32(1);int32(1);int32(1);int32(1);int32(1);int32(1);int32(1);int32(1);int32(1)]')  MultiplexValues=str2num('[double(0);double(0);double(0);double(0);double(0);double(0);double(0);double(0);double(0);double(0);double(0);double(0);double(0);double(0);double(0);double(0);double(0);double(0);double(0)]')  Factors=str2num('[double(1);double(1);double(1);double(1);double(1);double(1);double(1);double(1);double(1);double(1);double(1);double(1);double(1);double(1);double(1);double(1);double(1);double(1);double(1)]')  Offsets=str2num('[double(0);double(0);double(0);double(0);double(0);double(0);double(0);double(0);double(0);double(0);double(0);double(0);double(0);double(0);double(0);double(0);double(0);double(0);double(0)]')  Minimums=str2num('[double(0);double(0);double(0);double(0);double(0);double(0);double(0);double(0);double(0);double(0);double(0);double(0);double(0);double(0);double(0);double(0);double(0);double(0);double(0)]')  Maximums=str2num('[double(1);double(1);double(1);double(1);double(1);double(1);double(1);double(1);double(1);double(31);double(1);double(5);double(1);double(1);double(1);double(1);double(1);double(15);double(1)]')  Remote=off
      settings: DataFormat=CANdb specified signals
  CAN Transmit5 : canlib/CAN Transmit  BlockHandle=18477.0001  DeviceMenu=Vector Virtual 1 (Channel 1)  Device=Vector Virtual 1 (Channel 1)  ObjConstructor=canChannel('Vector', 'Virtual 1', 1)  EnablePeriodicTransmit=off  MessagePeriod=1.000
  Data Type Conversion1 : DataTypeConversion
  Ground_{1..18} (18 alike) : Ground
  Mux : Mux  Inputs=2
  Rate Transition : RateTransition
  Rate Transition1 : RateTransition
  wires:
  MABx/1 -> Bus Selector1/1, Bus Selector3/1
  Data Type Conversion1/1 -> Rate Transition/1  "Mode"
  CAN Pack5/1 -> Mux/1
  Bus Selector3/1 -> Data Type Conversion1/1  "<Mode>"
  Rate Transition/1 -> CAN Pack5/18
  Ground_1/1 -> CAN Pack5/1
  Ground_2/1 -> CAN Pack5/2
  Ground_3/1 -> CAN Pack5/3
  Ground_4/1 -> CAN Pack5/4
  Ground_5/1 -> CAN Pack5/5
  Ground_6/1 -> CAN Pack5/6
  Ground_7/1 -> CAN Pack5/7
  Ground_8/1 -> CAN Pack5/8
  Ground_9/1 -> CAN Pack5/9
  Ground_10/1 -> CAN Pack5/10
  Ground_11/1 -> CAN Pack5/11
  Ground_12/1 -> CAN Pack5/12
  Ground_13/1 -> CAN Pack5/13
  Ground_15/1 -> CAN Pack5/15
  Ground_16/1 -> CAN Pack5/16
  Ground_17/1 -> CAN Pack5/17
  Ground_18/1 -> CAN Pack5/19
  Bus Selector3/2 -> Rate Transition1/1  "<Shift_In_Progress>"
  Rate Transition1/1 -> CAN Pack5/14
  Bus Selector1/1 -> CAN Pack1/2  "<LowVoltEnblRq>"
  Bus Selector1/2 -> CAN Pack1/3  "<LwVltStpntCmnd>"
  Bus Selector1/3 -> CAN Pack1/4  "<PrplsnSysAtv>"
  Ground_14/1 -> CAN Pack1/1
  CAN Pack1/1 -> Mux/2
  Mux/1 -> CAN Transmit5/1

== system EcoSIM3_P2_C2_WIP/Powertrain/Clutch_Transmission2/Trans_Plant/Plant/Gear1-2/PI ==
  Actual_Pos : Inport
  Desired_Pos : Inport  Port=2
  I : Constant  Value=0
  Integrator1 : Integrator
  P : Constant  Value=3
  Product3 : Product  RndMeth=Zero
  Product4 : Product  RndMeth=Zero
  Saturation : Saturate  UpperLimit=10  LowerLimit=-10
  Sum3 : Sum  Inputs=|-+  SaturateOnIntegerOverflow=on  InputSameDT=on  OutDataTypeStr=Inherit: Same as first input
  Sum4 : Sum  SaturateOnIntegerOverflow=on  InputSameDT=on  OutDataTypeStr=Inherit: Same as first input
  Sum5 : Sum  Inputs=|+-  SaturateOnIntegerOverflow=on  InputSameDT=on  OutDataTypeStr=Inherit: Same as first input
  Force : Outport
  wires:
  Product3/1 -> Sum4/2
  Product4/1 -> Sum4/1
  Integrator1/1 -> Product3/1
  Sum3/1 -> Integrator1/1
  P/1 -> Product4/1
  Sum5/1 -> Product4/2
  I/1 -> Product3/2
  Saturation/1 -> Force/1
  Sum4/1 -> Saturation/1
  Desired_Pos/1 -> Sum3/2, Sum5/1
  Actual_Pos/1 -> Sum3/1, Sum5/2

== system EcoSIM3_P2_C2_WIP/Powertrain/Clutch_Transmission2/Trans_Plant/Plant/Gear1-2/Shaft Position ==
  Position_mm : Inport
  Add : Sum  Inputs=+++
  Compare To Constant : simulink/Logic and Bit Operations/Compare To Constant  relop=>=  const=0.05  OutDataTypeStr=boolean
  Data Type Conversion{,1..3} (4 alike) : DataTypeConversion
  Gain2 : Gain  Gain=3
  Gain3 : Gain  Gain=2
  Gain4 : Gain
  Integrator : Integrator  ExternalReset=either
  Interval Test : simulink/Logic and Bit Operations/Interval Test  IntervalClosedRight=on  uplimit=inf  IntervalClosedLeft=on  lowlimit=2.5  OutDataTypeStr=boolean
  Interval Test1 : simulink/Logic and Bit Operations/Interval Test  IntervalClosedRight=on  uplimit=1  IntervalClosedLeft=on  lowlimit=-1  OutDataTypeStr=boolean
  Interval Test2 : simulink/Logic and Bit Operations/Interval Test  IntervalClosedRight=on  uplimit=-2.5  IntervalClosedLeft=on  lowlimit=-inf  OutDataTypeStr=boolean
  Position : Outport
  wires:
  Position_mm/1 -> Interval Test2/1, Interval Test/1, Interval Test1/1
  Interval Test/1 -> Data Type Conversion/1
  Interval Test1/1 -> Data Type Conversion1/1
  Interval Test2/1 -> Data Type Conversion2/1
  Data Type Conversion2/1 -> Gain4/1
  Data Type Conversion/1 -> Gain2/1
  Gain4/1 -> Add/3
  Gain3/1 -> Add/2
  Gain2/1 -> Add/1
  Add/1 -> Position/1
  Integrator/1 -> Compare To Constant/1
  Compare To Constant/1 -> Data Type Conversion3/1
  Data Type Conversion3/1 -> Gain3/1
  Data Type Conversion1/1 -> Integrator/1, Integrator/2

== system EcoSIM3_P2_C2_WIP/Powertrain/Clutch_Transmission2/Trans_Plant/Plant/Gear3-4/PI2 ==
  Actual_Pos : Inport
  Desired_Pos : Inport  Port=2
  I : Constant  Value=0
  Integrator1 : Integrator
  P : Constant  Value=3
  Product3 : Product  RndMeth=Zero
  Product4 : Product  RndMeth=Zero
  Saturation : Saturate  UpperLimit=10  LowerLimit=-10
  Sum3 : Sum  Inputs=|-+  SaturateOnIntegerOverflow=on  InputSameDT=on  OutDataTypeStr=Inherit: Same as first input
  Sum4 : Sum  SaturateOnIntegerOverflow=on  InputSameDT=on  OutDataTypeStr=Inherit: Same as first input
  Sum5 : Sum  Inputs=|+-  SaturateOnIntegerOverflow=on  InputSameDT=on  OutDataTypeStr=Inherit: Same as first input
  Force : Outport
  wires:
  Saturation/1 -> Force/1
  I/1 -> Product3/2
  Sum5/1 -> Product4/2
  P/1 -> Product4/1
  Sum3/1 -> Integrator1/1
  Integrator1/1 -> Product3/1
  Product4/1 -> Sum4/1
  Product3/1 -> Sum4/2
  Sum4/1 -> Saturation/1
  Desired_Pos/1 -> Sum5/1, Sum3/2
  Actual_Pos/1 -> Sum5/2, Sum3/1

== system EcoSIM3_P2_C2_WIP/Powertrain/Clutch_Transmission2/Trans_Plant/Plant/Gear3-4/Shaft Position ==
  Position_mm : Inport
  Add : Sum  Inputs=+++
  Compare To Constant : simulink/Logic and Bit Operations/Compare To Constant  relop=>=  const=0.05  OutDataTypeStr=boolean
  Data Type Conversion{,1..3} (4 alike) : DataTypeConversion
  Gain2 : Gain  Gain=3
  Gain3 : Gain  Gain=2
  Gain4 : Gain
  Integrator : Integrator  ExternalReset=either
  Interval Test : simulink/Logic and Bit Operations/Interval Test  IntervalClosedRight=on  uplimit=inf  IntervalClosedLeft=on  lowlimit=2.5  OutDataTypeStr=boolean
  Interval Test1 : simulink/Logic and Bit Operations/Interval Test  IntervalClosedRight=on  uplimit=1  IntervalClosedLeft=on  lowlimit=-1  OutDataTypeStr=boolean
  Interval Test2 : simulink/Logic and Bit Operations/Interval Test  IntervalClosedRight=on  uplimit=-2.5  IntervalClosedLeft=on  lowlimit=-inf  OutDataTypeStr=boolean
  Position : Outport
  wires:
  Position_mm/1 -> Interval Test2/1, Interval Test/1, Interval Test1/1
  Interval Test/1 -> Data Type Conversion/1
  Interval Test1/1 -> Data Type Conversion1/1
  Interval Test2/1 -> Data Type Conversion2/1
  Data Type Conversion1/1 -> Integrator/2, Integrator/1
  Data Type Conversion2/1 -> Gain4/1
  Data Type Conversion/1 -> Gain2/1
  Gain4/1 -> Add/3
  Gain3/1 -> Add/2
  Gain2/1 -> Add/1
  Add/1 -> Position/1
  Data Type Conversion3/1 -> Gain3/1
  Integrator/1 -> Compare To Constant/1
  Compare To Constant/1 -> Data Type Conversion3/1

== system EcoSIM3_P2_C2_WIP/Powertrain/Clutch_Transmission2/Trans_Plant/Plant/Gear5-R/PI2 ==
  Actual_Pos : Inport
  Desired_Pos : Inport  Port=2
  I : Constant  Value=0
  Integrator1 : Integrator
  P : Constant  Value=3
  Product3 : Product  RndMeth=Zero
  Product4 : Product  RndMeth=Zero
  Saturation : Saturate  UpperLimit=10  LowerLimit=-10
  Sum3 : Sum  Inputs=|-+  SaturateOnIntegerOverflow=on  InputSameDT=on  OutDataTypeStr=Inherit: Same as first input
  Sum4 : Sum  SaturateOnIntegerOverflow=on  InputSameDT=on  OutDataTypeStr=Inherit: Same as first input
  Sum5 : Sum  Inputs=|+-  SaturateOnIntegerOverflow=on  InputSameDT=on  OutDataTypeStr=Inherit: Same as first input
  Force : Outport
  wires:
  Actual_Pos/1 -> Sum3/1, Sum5/2
  Desired_Pos/1 -> Sum3/2, Sum5/1
  Sum4/1 -> Saturation/1
  Product3/1 -> Sum4/2
  Product4/1 -> Sum4/1
  Integrator1/1 -> Product3/1
  Sum3/1 -> Integrator1/1
  P/1 -> Product4/1
  Sum5/1 -> Product4/2
  I/1 -> Product3/2
  Saturation/1 -> Force/1

== system EcoSIM3_P2_C2_WIP/Powertrain/Clutch_Transmission2/Trans_Plant/Plant/Gear5-R/Shaft Position ==
  Position_mm : Inport
  Add : Sum  Inputs=+++
  Data Type Conversion : DataTypeConversion
  Data Type Conversion1 : DataTypeConversion
  Data Type Conversion2 : DataTypeConversion
  Gain2 : Gain  Gain=3
  Gain3 : Gain  Gain=2
  Gain4 : Gain
  Interval Test : simulink/Logic and Bit Operations/Interval Test  IntervalClosedRight=on  uplimit=inf  IntervalClosedLeft=on  lowlimit=2.5  OutDataTypeStr=boolean
  Interval Test1 : simulink/Logic and Bit Operations/Interval Test  IntervalClosedRight=on  uplimit=1  IntervalClosedLeft=on  lowlimit=-1  OutDataTypeStr=boolean
  Interval Test2 : simulink/Logic and Bit Operations/Interval Test  IntervalClosedRight=on  uplimit=-2.5  IntervalClosedLeft=on  lowlimit=-inf  OutDataTypeStr=boolean
  Position : Outport
  wires:
  Position_mm/1 -> Interval Test2/1, Interval Test/1, Interval Test1/1
  Interval Test/1 -> Data Type Conversion/1
  Interval Test1/1 -> Data Type Conversion1/1
  Interval Test2/1 -> Data Type Conversion2/1
  Data Type Conversion1/1 -> Gain3/1
  Data Type Conversion2/1 -> Gain4/1
  Data Type Conversion/1 -> Gain2/1
  Gain4/1 -> Add/3
  Gain3/1 -> Add/2
  Gain2/1 -> Add/1
  Add/1 -> Position/1
